simulink model "Practica1"  (R2025a)
settings: Solver=VariableStepAuto  StartTime=0.0  StopTime=10.0  RelTol=1e-3
undefined symbols (not defined in the file): Beq, Bp, Fc, g, Ip, lp, Mc, Mp

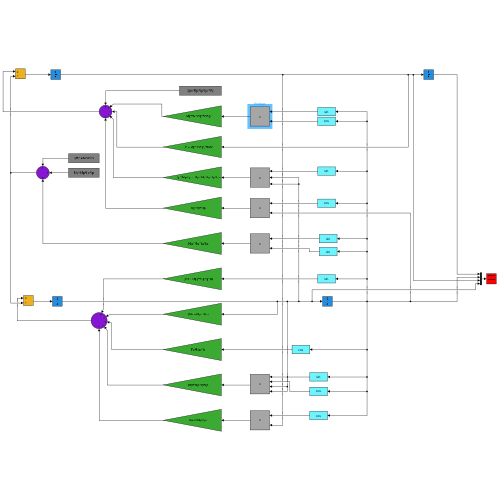
[thumbnail: Simulink's stored preview of the top-level diagram]
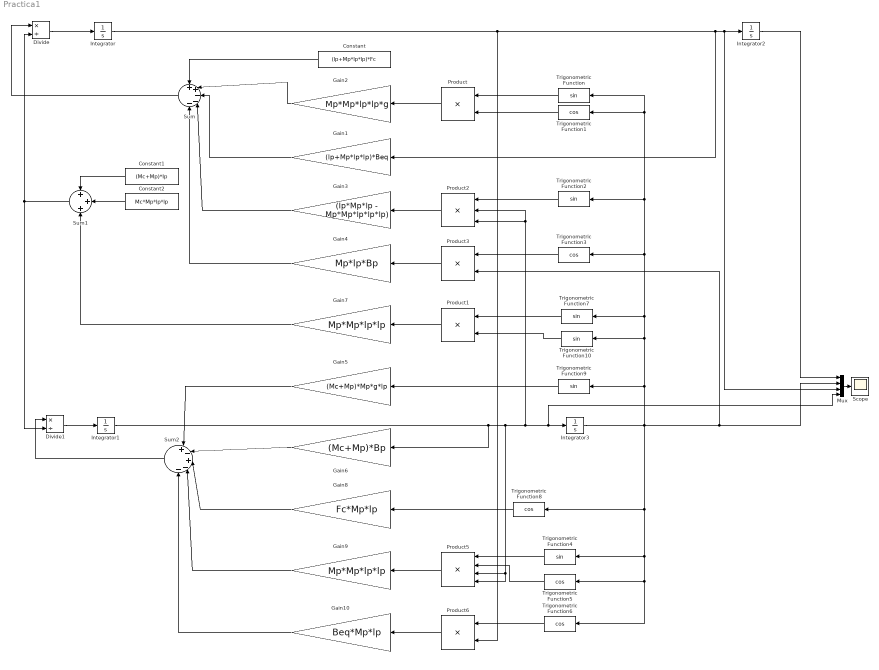
== system Practica1 ==
  Constant : Constant  Value=(lp+Mp*lp*lp)*Fc
  Constant1 : Constant  Value=(Mc+Mp)*Ip
  Constant2 : Constant  Value=Mc*Mp*lp*lp
  Divide : Product  Inputs=*/
  Divide1 : Product  Inputs=*/
  Gain1 : Gain  Gain=(lp+Mp*lp*lp)*Beq
  Gain10 : Gain  Gain=Beq*Mp*lp
  Gain2 : Gain  Gain=Mp*Mp*lp*lp*g
  Gain3 : Gain  Gain=(Ip*Mp*lp - Mp*Mp*lp*lp*lp)
  Gain4 : Gain  Gain=Mp*lp*Bp
  Gain5 : Gain  Gain=(Mc+Mp)*Mp*g*lp
  Gain6 : Gain  Gain=(Mc+Mp)*Bp
  Gain7 : Gain  Gain=Mp*Mp*lp*lp
  Gain8 : Gain  Gain=Fc*Mp*lp
  Gain9 : Gain  Gain=Mp*Mp*lp*lp
  Integrator : Integrator
  Integrator1 : Integrator
  Integrator2 : Integrator
  Integrator3 : Integrator  InitialCondition=pi/180
  Mux : Mux
  Product{,1,3,6} (4 alike) : Product
  Product2 : Product  Inputs=3
  Product5 : Product  Inputs=4
  Scope : Scope
      settings: ActiveDisplayYMinimum=-1.5137225464319275  ActiveDisplayYMaximum=1.8055732319617279
  Sum : Sum  Inputs=++---
  Sum1 : Sum  Inputs=+++
  Sum2 : Sum  Inputs=|+|-|+|-|-
  Trigonometric Function{,2,4,7,9..10} (6 alike) : Trigonometry
  Trigonometric Function{1,3,5..6,8} (5 alike) : Trigonometry  Operator=cos
  wires:
  Mux/1 -> Scope/1
  Divide/1 -> Integrator/1
  Integrator/1 -> Product6/2, Gain1/1, Mux/3, Integrator2/1
  Integrator2/1 -> Mux/1
  Divide1/1 -> Integrator1/1
  Integrator3/1 -> Trigonometric Function4/1, Trigonometric Function5/1, Trigonometric Function6/1, Trigonometric Function8/1, Trigonometric Function9/1, Trigonometric Function7/1, Trigonometric Function2/1, Trigonometric Function1/1, Trigonometric Function/1, Trigonometric Function3/1, Trigonometric Function10/1, Product3/2, Mux/2
  Product/1 -> Gain2/1
  Product2/1 -> Gain3/1
  Product3/1 -> Gain4/1
  Product1/1 -> Gain7/1
  Constant/1 -> Sum/1
  Gain2/1 -> Sum/2
  Gain1/1 -> Sum/3
  Gain3/1 -> Sum/4
  Gain4/1 -> Sum/5
  Trigonometric Function/1 -> Product/1
  Trigonometric Function1/1 -> Product/2
  Trigonometric Function2/1 -> Product2/1
  Integrator1/1 -> Gain6/1, Product5/3, Product5/4, Product2/3, Product2/2, Mux/4, Integrator3/1
  Trigonometric Function3/1 -> Product3/1
  Trigonometric Function7/1 -> Product1/1
  Trigonometric Function9/1 -> Gain5/1
  Trigonometric Function8/1 -> Gain8/1
  Product5/1 -> Gain9/1
  Trigonometric Function4/1 -> Product5/1
  Trigonometric Function5/1 -> Product5/2
  Product6/1 -> Gain10/1
  Trigonometric Function6/1 -> Product6/1
  Gain5/1 -> Sum2/1
  Gain6/1 -> Sum2/2
  Gain8/1 -> Sum2/3
  Gain9/1 -> Sum2/4
  Gain10/1 -> Sum2/5
  Constant1/1 -> Sum1/1
  Constant2/1 -> Sum1/2
  Gain7/1 -> Sum1/3
  Sum1/1 -> Divide1/2, Divide/2
  Sum/1 -> Divide/1
  Sum2/1 -> Divide1/1
  Trigonometric Function10/1 -> Product1/2
